simulink model "main"  (R2024a)
settings: Solver=VariableStepAuto  StartTime=0.0  StopTime=inf  RelTol=1e-3
libraries: vrlib x1
settings Model: Creator=jd632  LastModifiedBy=jd632
settings RTWCC: GPUComputeCapability=3.5

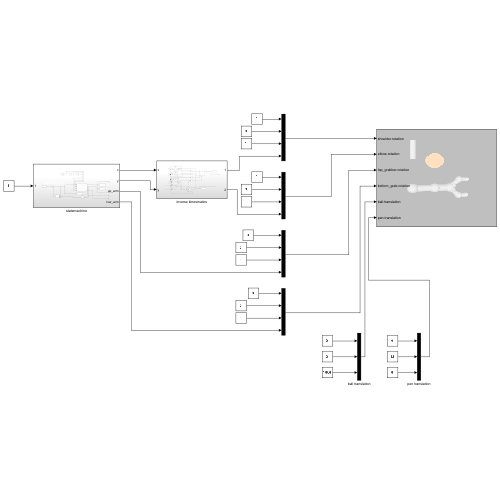
[thumbnail: Simulink's stored preview of the top-level diagram]
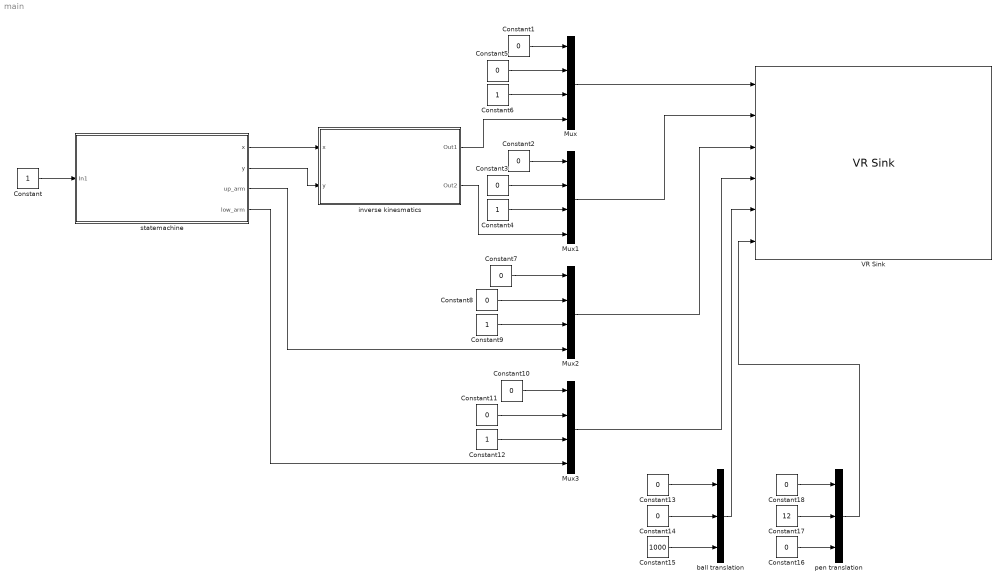
== system main ==
  Constant{,4,6,9,12} (5 alike) : Constant
  Constant{1..3,5,7..8,10..11,13..14,16,18} (12 alike) : Constant  Value=0
  Constant15 : Constant  Value=1000
  Constant17 : Constant  Value=12
  Mux{,1..3} (4 alike) : Mux
  VR Sink : vrlib/VR Sink  InstantiateOnLoad=on  SampleTime=0.1  ViewEnable=on  RemoteChange=off  RemoteView=off  FieldsWritten=shoulder.rotation.4.1.1.double#elbow.rotation.4.1.1.double#top_grabber.rotation.4.1.1.double#bottom_grab.rotation.4.1.1.double#ball.translation.3.1.1.double#pen.translation.3.1.1.double  WorldFileName=final_arm.wrl  AutoView=off  VideoDimensions=[]  AllowVariableSize=off
  ball translation : Mux  Inputs=3
  inverse kinesmatics : Subsystem
  pen translation : Mux  Inputs=3
  statemachine : Subsystem
  wires:
  Constant3/1 -> Mux1/2
  Constant5/1 -> Mux/2
  Constant2/1 -> Mux1/1
  Constant1/1 -> Mux/1
  Constant6/1 -> Mux/3
  Constant4/1 -> Mux1/3
  inverse kinesmatics/2(Out2) -> Mux1/4
  inverse kinesmatics/1(Out1) -> Mux/4
  statemachine/2(y) -> inverse kinesmatics/2(y)
  statemachine/1(x) -> inverse kinesmatics/1(x)
  Constant/1 -> statemachine/1(In1)
  statemachine/3(up_arm) -> Mux2/4
  statemachine/4(low_arm) -> Mux3/4
  Constant9/1 -> Mux2/3
  Constant7/1 -> Mux2/1
  Constant8/1 -> Mux2/2
  Constant11/1 -> Mux3/2
  Constant10/1 -> Mux3/1
  Constant12/1 -> Mux3/3
  Mux/1 -> VR Sink/1
  Mux1/1 -> VR Sink/2
  Mux2/1 -> VR Sink/3
  Mux3/1 -> VR Sink/4
  Constant18/1 -> pen translation/1
  Constant17/1 -> pen translation/2
  Constant16/1 -> pen translation/3
  pen translation/1 -> VR Sink/6
  Constant15/1 -> ball translation/3
  Constant14/1 -> ball translation/2
  Constant13/1 -> ball translation/1
  ball translation/1 -> VR Sink/5

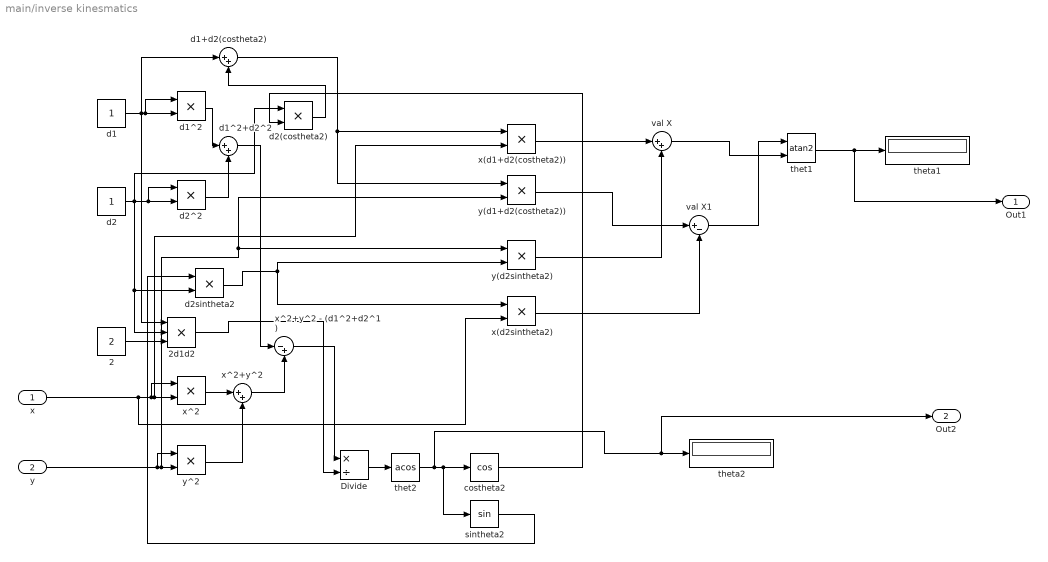
== system main/inverse kinesmatics ==
  x : Inport
  y : Inport  Port=2
  2 : Constant  Value=2
  2d1d2 : Product  Inputs=3
  Divide : Product  Inputs=*/
  costheta2 : Trigonometry  Operator=cos
  d1 : Constant
  d1+d2(costheta2) : Sum  Inputs=|++
  d1^2 : Product
  d1^2+d2^2 : Sum  Inputs=|++
  d2 : Constant
  d2(costheta2) : Product
  d2^2 : Product
  d2sintheta2 : Product
  sintheta2 : Trigonometry
  thet1 : Trigonometry  Operator=atan2
  thet2 : Trigonometry  Operator=acos
  theta1 : Display
  theta2 : Display
  val X : Sum  Inputs=|++
  val X1 : Sum  Inputs=|+-
  x(d1+d2(costheta2)) : Product
  x(d2sintheta2) : Product
  x^2 : Product
  x^2+y^2 : Sum  Inputs=|++
  x^2+y^2 - (d1^2+d2^1) : Sum  Inputs=|-+
  y(d1+d2(costheta2)) : Product
  y(d2sintheta2) : Product
  y^2 : Product
  Out1 : Outport
  Out2 : Outport  Port=2
  wires:
  thet2/1 -> Out2/1, theta2/1, sintheta2/1, costheta2/1
  d1^2/1 -> d1^2+d2^2/1
  x/1 -> x(d2sintheta2)/2, x(d1+d2(costheta2))/2, x^2/2, x^2/1
  thet1/1 -> Out1/1, theta1/1
  d2/1 -> d2(costheta2)/1, 2d1d2/2, d2sintheta2/2, d2^2/1, d2^2/2
  d2(costheta2)/1 -> d1+d2(costheta2)/2
  y/1 -> y(d1+d2(costheta2))/2, y(d2sintheta2)/1, y^2/2, y^2/1
  Divide/1 -> thet2/1
  x^2+y^2/1 -> x^2+y^2 - (d1^2+d2^1)/2
  d1^2+d2^2/1 -> x^2+y^2 - (d1^2+d2^1)/1
  d1+d2(costheta2)/1 -> y(d1+d2(costheta2))/1, x(d1+d2(costheta2))/1
  val X/1 -> thet1/2
  d1/1 -> d1+d2(costheta2)/1, 2d1d2/1, d1^2/1, d1^2/2
  2/1 -> 2d1d2/3
  val X1/1 -> thet1/1
  x(d2sintheta2)/1 -> val X1/2
  sintheta2/1 -> d2sintheta2/1
  2d1d2/1 -> Divide/2
  x^2+y^2 - (d1^2+d2^1)/1 -> Divide/1
  d2sintheta2/1 -> x(d2sintheta2)/1, y(d2sintheta2)/2
  x(d1+d2(costheta2))/1 -> val X/1
  y(d1+d2(costheta2))/1 -> val X1/1
  y(d2sintheta2)/1 -> val X/2
  d2^2/1 -> d1^2+d2^2/2
  x^2/1 -> x^2+y^2/1
  y^2/1 -> x^2+y^2/2
  costheta2/1 -> d2(costheta2)/2

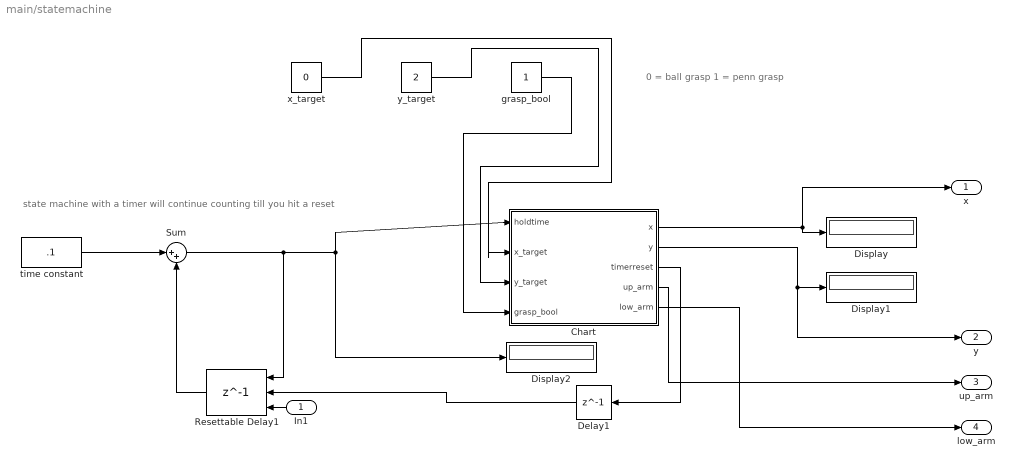
== system main/statemachine ==
  note: state machine with a timer will continue counting till you hit a reset
  note: 0 = ball grasp 1 = penn grasp
  In1 : Inport
  Chart : Stateflow chart  TreatAsAtomicUnit=on
  Delay1 : Delay  DelayLength=1  InitialCondition=0
  Display : Display
  Display1 : Display
  Display2 : Display
  Resettable Delay1 : Delay  DelayLength=1  InitialConditionSource=Input port  ExternalReset=Rising
      settings: InputPortMap=u0,r5,p4
  Sum : Sum  Inputs=|++
  grasp_bool : Constant
  time constant : Constant  Value=.1
  x_target : Constant  Value=0
  y_target : Constant  Value=2
  x : Outport
  y : Outport  Port=2
  up_arm : Outport  Port=3
  low_arm : Outport  Port=4
  wires:
  Resettable Delay1/1 -> Sum/2
  Delay1/1 -> Resettable Delay1/2
  In1/1 -> Resettable Delay1/3
  Sum/1 -> Resettable Delay1/1, Display2/1, Chart/1(holdtime)
  time constant/1 -> Sum/1
  Chart/3(timerreset) -> Delay1/1
  Chart/2(y) -> y/1, Display1/1
  Chart/1(x) -> Display/1, x/1
  x_target/1 -> Chart/2(x_target)
  y_target/1 -> Chart/3(y_target)
  grasp_bool/1 -> Chart/4(grasp_bool)
  Chart/4(up_arm) -> up_arm/1
  Chart/5(low_arm) -> low_arm/1

== stateflow chart main/statemachine/Chart ==
  state start
    x=0; y=0;
    up_arm = 1;
    low_arm = -1;
    timerreset = 0;
  state centerstate
    x=0; y=0;up_arm = 1;
    low_arm = -1;
    timerreset =0;
  state resetimerstate
    x=0; y=0;
    timerreset = 1;
  state move_x
    x=x+0.001; y =0;
    up_arm = 1; low_arm =-1;
    timerreset = 0;
  state centerstateback
    x=0; y=0;
    timerreset = 0;
  state move_y_center
    x=0; y= y-0.001;
    timerreset = 0;
  state move_y
    x = x_target; y=y+0.001;
    up_arm =1;
    low_arm = -1;
    timerreset = 0;
  state move_x_center
    x=x-0.001; y= y_target;
    timerreset = 0;
  state at_target
    x=x_target; y=y_target;
    up_arm =1; low_arm =-1;
    timerreset = 0;
  state grasp_pen_state
    x = x_target; y = y_target;
    up_arm = up_arm - 0.001; low_arm = low_arm +0.001;
    timerreset = 0;
  state grasp_ball_state
    x = x_target; y = y_target;
    up_arm = up_arm - 0.001; low_arm = low_arm +0.001;
    timerreset = 0;
  (default) -> start
  start -> centerstate
  resetimerstate -> centerstate
  centerstateback -> resetimerstate : [holdtime > 75]
  centerstate -> move_x : [holdtime > 25]
  move_x -> move_y : [x>= x_target]
  move_y_center -> centerstateback : [y <= 0]
  move_x_center -> move_y_center : [x<=0]
  move_y -> at_target : [y >= y_target]
  grasp_pen_state -> move_x_center : [up_arm <= .5 && low_arm >= -.5]
  grasp_ball_state -> move_x_center : [up_arm <= .75 && low_arm >= -.75]
  at_target -> grasp_pen_state [order 2] : [grasp_bool ==1]
  at_target -> grasp_ball_state [order 1] : [grasp_bool == 0]
  data: holdtime input; x output; y output; timerreset output; x_target input [0..2]; y_target input [0..2]; grasp_bool input [0..1]; up_arm output; low_arm output
